simulink model "HDVPSG_DelayComp_NewRef_RealDrop_case1"  (R2019b)
settings: Solver=FixedStepDiscrete  StartTime=0.0  StopTime=28  FixedStep=UT.Ts_Veh  RelTol=1e-3
PostLoadFcn:
  | if any(exist('dsrtsu_mdlpostloadfcn', 'file') ~= 0), dsrtsu_mdlpostloadfcn('Execute', bdroot); end
InitFcn:
  | , if any(exist('dsmpb_private', 'file') ~= 0), dsmpb_private('dsmpb_mdlclblib', 'Init', bdroot); end,
values from neighbouring files (symbols this model uses):
  BETA_HDV_Leader = 50    [HDVPSG_DelayComp_NewRef_RealDrop_script_case1.m]
  BETA_PSG_Follower = 150    [HDVPSG_DelayComp_NewRef_RealDrop_script_case1.m]
  CtrlZone_Length = 250    [HDVPSG_DelayComp_NewRef_RealDrop_script_case1.m]
  DELTA_D_MIN = 5    [HDVPSG_DelayComp_NewRef_RealDrop_script_case1.m]
  DELTA_DR_MG_TCC = 15    [HDVPSG_DelayComp_NewRef_RealDrop_script_case1.m]
  HDV_AMAX = 1.3    [HDVPSG_DelayComp_NewRef_RealDrop_script_case1.m]
  HDV_AMIN = -2.5    [HDVPSG_DelayComp_NewRef_RealDrop_script_case1.m]
  HDV_first_v0 = 13    [HDVPSG_DelayComp_NewRef_RealDrop_script_case1.m]
  HDV_HighMu_D = 9    [HDVPSG_DelayComp_NewRef_RealDrop_script_case1.m]
  HDV_HighMu_I = 27    [HDVPSG_DelayComp_NewRef_RealDrop_script_case1.m]
  HDV_HighMu_P = 27    [HDVPSG_DelayComp_NewRef_RealDrop_script_case1.m]
  HDV_HighMu_TRFC = 0.7    [HDVPSG_DelayComp_NewRef_RealDrop_script_case1.m]
  HDV_last_v0 = 13    [HDVPSG_DelayComp_NewRef_RealDrop_script_case1.m]
  HDV_LowMu_D = 6    [HDVPSG_DelayComp_NewRef_RealDrop_script_case1.m]
  HDV_LowMu_I = 8    [HDVPSG_DelayComp_NewRef_RealDrop_script_case1.m]
  HDV_LowMu_P = 12    [HDVPSG_DelayComp_NewRef_RealDrop_script_case1.m]
  HDV_LowMu_TRFC = 0.6    [HDVPSG_DelayComp_NewRef_RealDrop_script_case1.m]
  Np_MPC = 20    [HDVPSG_DelayComp_NewRef_RealDrop_script_case1.m]
  PSG_AMAX = 3.2    [HDVPSG_DelayComp_NewRef_RealDrop_script_case1.m]
  PSG_AMIN = -6    [HDVPSG_DelayComp_NewRef_RealDrop_script_case1.m]
  PSG_end_v0 = 13    [HDVPSG_DelayComp_NewRef_RealDrop_script_case1.m]
  PSG_first_v0 = 13    [HDVPSG_DelayComp_NewRef_RealDrop_script_case1.m]
  PSG_HighMu_D = 15    [HDVPSG_DelayComp_NewRef_RealDrop_script_case1.m]
  PSG_HighMu_I = 125    [HDVPSG_DelayComp_NewRef_RealDrop_script_case1.m]
  PSG_HighMu_P = 75    [HDVPSG_DelayComp_NewRef_RealDrop_script_case1.m]
  PSG_HighMu_TRFC = 0.8    [HDVPSG_DelayComp_NewRef_RealDrop_script_case1.m]
  PSG_LowMu_D = 12    [HDVPSG_DelayComp_NewRef_RealDrop_script_case1.m]
  PSG_LowMu_I = 64    [HDVPSG_DelayComp_NewRef_RealDrop_script_case1.m]
  PSG_LowMu_P = 48    [HDVPSG_DelayComp_NewRef_RealDrop_script_case1.m]
  PSG_LowMu_TRFC = 0.7    [HDVPSG_DelayComp_NewRef_RealDrop_script_case1.m]
  PSG_middle_v0 = 13    [HDVPSG_DelayComp_NewRef_RealDrop_script_case1.m]
  Q_Leader = 1    [HDVPSG_DelayComp_NewRef_RealDrop_script_case1.m]
  Qd_dot_PSG_Follower = 2    [HDVPSG_DelayComp_NewRef_RealDrop_script_case1.m]
  Qd_PSG_Follower = 10    [HDVPSG_DelayComp_NewRef_RealDrop_script_case1.m]
  R_Leader = 20    [HDVPSG_DelayComp_NewRef_RealDrop_script_case1.m]
  R_PSG_Follower = 1    [HDVPSG_DelayComp_NewRef_RealDrop_script_case1.m]
  Recved_40_1 = Recved_Flag_Combined(47740,:)    [HDVPSG_DelayComp_NewRef_RealDrop_script_case1.m]
  Recved_40_2 = Recved_Flag_Combined(47780,:)    [HDVPSG_DelayComp_NewRef_RealDrop_script_case1.m]
  Recved_40_3 = Recved_Flag_Combined(49536,:)    [HDVPSG_DelayComp_NewRef_RealDrop_script_case1.m]
  Recved_40_4 = Recved_Flag_Combined(118106,:)    [HDVPSG_DelayComp_NewRef_RealDrop_script_case1.m]
  Rho_deltad_PSG_Follower = 1e3    (= 1000)    [HDVPSG_DelayComp_NewRef_RealDrop_script_case1.m]
  Rho_v_PSG_Follower = 1e3    (= 1000)    [HDVPSG_DelayComp_NewRef_RealDrop_script_case1.m]
  T_ADE = 0.01    [HDVPSG_DelayComp_NewRef_RealDrop_script_case1.m]
  V_MAX = 40    [HDVPSG_DelayComp_NewRef_RealDrop_script_case1.m]
  V_MIN = 0    [HDVPSG_DelayComp_NewRef_RealDrop_script_case1.m]
  VR_MG_TCC = 15    [HDVPSG_DelayComp_NewRef_RealDrop_script_case1.m]
undefined symbols (not defined in the file or in its folder): DiscIntNeverNeededParam, UT
libraries: simulink x46
(part 14 of 16)

== system HDVPSG_DelayComp_NewRef_RealDrop_case1/Subsystem6/HDV_first/Body Fixed Vehicle Dynamics/8dof_vehicle/longitudinal ==
  In1 : Inport
  In2 : Inport  Port=2
  In5 : Inport  Port=3
  In6 : Inport  Port=4
  In3 : Inport  Port=5
  In4 : Inport  Port=6
  Fax : Inport  Port=7
  Fr : Inport  Port=8
  slope : Inport  Port=9
  Vy : Inport  Port=10
  deltaFL : Inport  Port=11
  deltaFR : Inport  Port=12
  pitch : Inport  Port=13
  pitch_rate : Inport  Port=14
  pitch_accel : Inport  Port=15
  roll : Inport  Port=16
  roll_rate : Inport  Port=17
  roll_accel : Inport  Port=18
  yaw_rate : Inport  Port=19
  yaw_accel : Inport  Port=20
  V_ini : Inport  Port=21
  Add : Sum  Inputs=+-++---
  Add1 : Sum  Inputs=+++
  Add2 : Sum
  Add3 : Sum  Inputs=+++
  Add4 : Sum
  Add5 : Sum  Inputs=+---++
  Constant : Constant  Value=UT.Mv
  Constant1 : Constant  Value=UT.g
  Discrete-Time Integrator : DiscreteIntegrator  InitialConditionSource=external  InitialCondition=UT.Veh_PSG_o(1)  SampleTime=UT.Ts_Veh  ICPrevOutput=DiscIntNeverNeededParam  ICPrevScaledInput=DiscIntNeverNeededParam
  Gain : Gain  Gain=1/UT.Mv
  Gain1 : Gain  Gain=UT.h
  Gain2 : Gain
  Gain3 : Gain  Gain=2
  Gain4 : Gain  Gain=2
  Math Function : Math  Operator=square  SaturateOnIntegerOverflow=on
  Math Function1 : Math  Operator=square  SaturateOnIntegerOverflow=on
  Math Function2 : Math  Operator=square  SaturateOnIntegerOverflow=on
  Product{,1..2,4..5,7} (6 alike) : Product
  Product10 : Product  Inputs=4
  Product{3,6,8..9,11} (5 alike) : Product  Inputs=3
  Saturation : Saturate  UpperLimit=50  LowerLimit=0
  Trigonometric {,3,6..7} (4 alike) : Trigonometry  Operator=cos
  Trigonometric {1..2,4..5,8} (5 alike) : Trigonometry
  yaw_rate1 : InportShadow  Port=19
  ax : Outport  VectorParamsAs1DForOutWhenUnconnected=off
  Vx : Outport  Port=2  VectorParamsAs1DForOutWhenUnconnected=off
  Fx : Outport  Port=3  VectorParamsAs1DForOutWhenUnconnected=off
  wires:
  Add5/1 -> Gain1/1
  roll_accel/1 -> Product11/3
  Product11/1 -> Add5/6
  Trigonometric 8/1 -> Product10/2, Product11/1
  Product10/1 -> Gain4/1
  Gain4/1 -> Add5/5
  Product9/1 -> Add5/4
  pitch_accel/1 -> Product9/3
  Trigonometric 7/1 -> Product9/2, Product10/1
  Gain3/1 -> Add5/3
  Product8/1 -> Gain3/1
  Product7/1 -> Add5/2
  yaw_accel/1 -> Product7/2
  Product6/1 -> Add5/1
  Trigonometric 5/1 -> Product6/1, Product11/2, Product7/1
  Trigonometric 6/1 -> Product6/2, Product8/1, Product9/1
  roll/1 -> Trigonometric 6/1, Trigonometric 8/1
  pitch/1 -> Trigonometric 5/1, Trigonometric 7/1
  Add3/1 -> Product6/3
  Math Function2/1 -> Add3/3
  Math Function1/1 -> Add3/2
  Math Function/1 -> Add3/1
  yaw_rate/1 -> Math Function2/1, Product8/3
  roll_rate/1 -> Math Function1/1, Product8/2, Product10/3
  pitch_rate/1 -> Math Function/1, Product10/4
  Gain1/1 -> Add1/3
  Saturation/1 -> Vx/1
  Product5/1 -> Add2/2
  Product2/1 -> Add2/1
  Trigonometric 4/1 -> Product5/2
  Trigonometric 1/1 -> Product2/2
  Trigonometric 3/1 -> Product1/2
  deltaFR/1 -> Trigonometric 3/1, Trigonometric 4/1
  "Trigonometric "/1 -> Product4/2
  deltaFL/1 -> "Trigonometric "/1, Trigonometric 1/1
  In2/1 -> Product1/1
  Product1/1 -> Add4/2
  Gain2/1 -> Add/6
  Constant/1 -> Product3/2
  Constant1/1 -> Product3/1
  Trigonometric 2/1 -> Product3/3
  Add1/1 -> ax/1, Discrete-Time Integrator/1
  In6/1 -> Add/4
  In5/1 -> Add/3
  Add2/1 -> Add/2
  In4/1 -> Product5/1
  In3/1 -> Product2/1
  Add4/1 -> Add/1
  Product4/1 -> Add4/1
  In1/1 -> Product4/1
  Gain/1 -> Add1/1
  Product/1 -> Add1/2
  Add/1 -> Gain/1, Fx/1
  Vy/1 -> Product/2
  yaw_rate1/1 -> Product/1
  Product3/1 -> Add/7
  slope/1 -> Trigonometric 2/1
  Fr/1 -> Gain2/1
  Fax/1 -> Add/5
  Discrete-Time Integrator/1 -> Saturation/1
  V_ini/1 -> Discrete-Time Integrator/2

== system HDVPSG_DelayComp_NewRef_RealDrop_case1/Subsystem6/HDV_first/Body Fixed Vehicle Dynamics/Driving Resistance Subsystem/Aerodynamic Resistance ==
  note: increaesd to 0.75*...
  note: Vx=m/s
  note: Fa=0.5*p*Cd*A(Vx+Vw)^2
  Vx : Inport
  X Aerodynamic Fcn : Fcn  Expr=0.75*UT.rho*UT.Cd*UT.Awind*(u(1)+UT.Vw)^2  SampleTime=UT.Ts_Veh
  Fa : Outport  VectorParamsAs1DForOutWhenUnconnected=off
  wires:
  Vx/1 -> X Aerodynamic Fcn/1
  X Aerodynamic Fcn/1 -> Fa/1

== system HDVPSG_DelayComp_NewRef_RealDrop_case1/Subsystem6/HDV_first/Body Fixed Vehicle Dynamics/Driving Resistance Subsystem/Rolling resistance ==
  note: added *2
  Vx : Inport
  Rolling resistance Fcn1 : Fcn  Expr=(0.005+(1/2.013)*(0.01+0.0095*((3.6*u(1))/100)^2))*UT.Mv*UT.g*2  SampleTime=UT.Ts_Veh
  Fr : Outport  VectorParamsAs1DForOutWhenUnconnected=off
  wires:
  Rolling resistance Fcn1/1 -> Fr/1
  Vx/1 -> Rolling resistance Fcn1/1

== system HDVPSG_DelayComp_NewRef_RealDrop_case1/Subsystem6/HDV_first/Body Fixed Vehicle Dynamics/Fz/FZ FL ==
  note: 0.5
  ax : Inport
  slope : Inport  Port=2
  ay : Inport  Port=3
  bank : Inport  Port=4
  Fa : Inport  Port=5
  Add1 : Sum  Inputs=--+-+-+
  Constant : Constant  Value=UT.ha
  Constant1 : Constant  Value=UT.Ms
  Constant{3,10,17,23} (4 alike) : Constant  Value=UT.g
  Constant11 : Constant  Value=UT.lf+UT.lr
  Constant{8,12,15,20} (4 alike) : Constant  Value=UT.Mv
  Constant{2,6,9,13} (4 alike) : Constant  Value=UT.h
  Constant14 : Constant  Value=2*UT.Ls
  Constant16 : Constant  Value=UT.lr
  Constant18 : Constant  Value=UT.lf +UT.lr
  Constant19 : Constant  Value=UT.lf+UT.lr
  Constant21 : Constant  Value=UT.Ls
  Constant22 : Constant  Value=2*UT.Ls
  Constant4 : Constant  Value=UT.lf+UT.lr
  Constant5 : Constant  Value=UT.Ms
  Constant7 : Constant  Value=2*UT.Ls
  Divide{,1..6} (7 alike) : Product  Inputs=*/
  Gain{,1..6} (7 alike) : Gain  Gain=0.25
  Product : Product
  Product1 : Product  Inputs=3
  Product{2,4..6} (4 alike) : Product  Inputs=4
  Product3 : Product  Inputs=3
  Trigonometric Function : Trigonometry
  Trigonometric Function1 : Trigonometry
  Trigonometric Function2 : Trigonometry  Operator=cos
  Trigonometric Function3 : Trigonometry  Operator=cos
  bank1 : InportShadow  Port=4
  slope1 : InportShadow  Port=2
  Out1 : Outport  VectorParamsAs1DForOutWhenUnconnected=off
  wires:
  Gain6/1 -> Add1/7
  Divide6/1 -> Gain6/1
  Constant22/1 -> Divide6/2
  Product6/1 -> Divide6/1
  Trigonometric Function3/1 -> Product6/4
  bank1/1 -> Trigonometric Function3/1
  Constant23/1 -> Product6/3
  Constant21/1 -> Product6/2
  Constant20/1 -> Product6/1
  Gain2/1 -> Add1/6
  Gain4/1 -> Add1/3
  Gain3/1 -> Add1/5
  Gain1/1 -> Add1/4
  Gain/1 -> Add1/2
  Gain5/1 -> Add1/1
  Divide5/1 -> Gain5/1
  Constant19/1 -> Divide5/2
  Product/1 -> Divide5/1
  Constant/1 -> Product/2
  Fa/1 -> Product/1
  Product1/1 -> Divide/1
  Add1/1 -> Out1/1
  Divide4/1 -> Gain3/1
  Product5/1 -> Divide4/1
  Constant18/1 -> Divide4/2
  slope1/1 -> Trigonometric Function2/1
  Trigonometric Function2/1 -> Product5/4
  Constant17/1 -> Product5/3
  Constant16/1 -> Product5/2
  Constant15/1 -> Product5/1
  Divide3/1 -> Gain2/1
  Constant14/1 -> Divide3/2
  Product2/1 -> Divide3/1
  Trigonometric Function1/1 -> Product2/4
  bank/1 -> Trigonometric Function1/1
  Constant3/1 -> Product2/3
  Constant13/1 -> Product2/2
  Constant12/1 -> Product2/1
  Product4/1 -> Divide2/1
  Divide2/1 -> Gain1/1
  Constant11/1 -> Divide2/2
  Trigonometric Function/1 -> Product4/4
  slope/1 -> Trigonometric Function/1
  Constant10/1 -> Product4/3
  Constant9/1 -> Product4/2
  Constant8/1 -> Product4/1
  Divide1/1 -> Gain4/1
  Divide/1 -> Gain/1
  Constant7/1 -> Divide1/2
  Product3/1 -> Divide1/1
  Constant6/1 -> Product3/3
  Constant5/1 -> Product3/2
  ay/1 -> Product3/1
  Constant4/1 -> Divide/2
  ax/1 -> Product1/3
  Constant2/1 -> Product1/2
  Constant1/1 -> Product1/1

== system HDVPSG_DelayComp_NewRef_RealDrop_case1/Subsystem6/HDV_first/Body Fixed Vehicle Dynamics/Fz/FZ FR ==
  note: 0.5
  ax : Inport
  slope : Inport  Port=2
  ay : Inport  Port=3
  bank : Inport  Port=4
  Fa : Inport  Port=5
  Add1 : Sum  Inputs=----+++
  Constant : Constant  Value=UT.ha
  Constant1 : Constant  Value=UT.Ms
  Constant{3,10,17,23} (4 alike) : Constant  Value=UT.g
  Constant{4,11,18..19} (4 alike) : Constant  Value=UT.lf+UT.lr
  Constant{8,12,15,20} (4 alike) : Constant  Value=UT.Mv
  Constant{2,6,9,13} (4 alike) : Constant  Value=UT.h
  Constant14 : Constant  Value=2*UT.Ls
  Constant16 : Constant  Value=UT.lr
  Constant21 : Constant  Value=UT.Ls
  Constant22 : Constant  Value=2*UT.Ls
  Constant5 : Constant  Value=UT.Ms
  Constant7 : Constant  Value=2*UT.Ls
  Divide{,1..6} (7 alike) : Product  Inputs=*/
  Gain{,1..6} (7 alike) : Gain  Gain=0.25
  Product : Product
  Product1 : Product  Inputs=3
  Product{2,4..6} (4 alike) : Product  Inputs=4
  Product3 : Product  Inputs=3
  Trigonometric Function : Trigonometry
  Trigonometric Function1 : Trigonometry
  Trigonometric Function2 : Trigonometry  Operator=cos
  Trigonometric Function3 : Trigonometry  Operator=cos
  bank1 : InportShadow  Port=4
  slope1 : InportShadow  Port=2
  Out1 : Outport  VectorParamsAs1DForOutWhenUnconnected=off
  wires:
  Constant1/1 -> Product1/1
  Constant2/1 -> Product1/2
  ax/1 -> Product1/3
  Constant4/1 -> Divide/2
  ay/1 -> Product3/1
  Constant5/1 -> Product3/2
  Constant6/1 -> Product3/3
  Product3/1 -> Divide1/1
  Constant7/1 -> Divide1/2
  Divide/1 -> Gain/1
  Divide1/1 -> Gain4/1
  Constant8/1 -> Product4/1
  Constant9/1 -> Product4/2
  Constant10/1 -> Product4/3
  slope/1 -> Trigonometric Function/1
  Trigonometric Function/1 -> Product4/4
  Constant11/1 -> Divide2/2
  Divide2/1 -> Gain1/1
  Product4/1 -> Divide2/1
  Constant12/1 -> Product2/1
  Constant13/1 -> Product2/2
  Constant3/1 -> Product2/3
  bank/1 -> Trigonometric Function1/1
  Trigonometric Function1/1 -> Product2/4
  Product2/1 -> Divide3/1
  Constant14/1 -> Divide3/2
  Divide3/1 -> Gain2/1
  Constant15/1 -> Product5/1
  Constant16/1 -> Product5/2
  Constant17/1 -> Product5/3
  Trigonometric Function2/1 -> Product5/4
  slope1/1 -> Trigonometric Function2/1
  Constant18/1 -> Divide4/2
  Product5/1 -> Divide4/1
  Divide4/1 -> Gain3/1
  Add1/1 -> Out1/1
  Product1/1 -> Divide/1
  Fa/1 -> Product/1
  Constant/1 -> Product/2
  Product/1 -> Divide5/1
  Constant19/1 -> Divide5/2
  Divide5/1 -> Gain5/1
  Gain5/1 -> Add1/1
  Gain/1 -> Add1/2
  Gain1/1 -> Add1/4
  Gain3/1 -> Add1/5
  Gain4/1 -> Add1/3
  Gain2/1 -> Add1/6
  Constant20/1 -> Product6/1
  Constant21/1 -> Product6/2
  Constant23/1 -> Product6/3
  bank1/1 -> Trigonometric Function3/1
  Trigonometric Function3/1 -> Product6/4
  Product6/1 -> Divide6/1
  Constant22/1 -> Divide6/2
  Divide6/1 -> Gain6/1
  Gain6/1 -> Add1/7

== system HDVPSG_DelayComp_NewRef_RealDrop_case1/Subsystem6/HDV_first/Body Fixed Vehicle Dynamics/Fz/FZ RL ==
  note: 0.5
  ax : Inport
  slope : Inport  Port=2
  ay : Inport  Port=3
  bank : Inport  Port=4
  Fa : Inport  Port=5
  Add1 : Sum  Inputs=+++++-+
  Constant : Constant  Value=UT.ha
  Constant1 : Constant  Value=UT.Ms
  Constant{3,10,17,23} (4 alike) : Constant  Value=UT.g
  Constant{4,11,18..19} (4 alike) : Constant  Value=UT.lf+UT.lr
  Constant{8,12,15,20} (4 alike) : Constant  Value=UT.Mv
  Constant{2,6,9,13} (4 alike) : Constant  Value=UT.h
  Constant14 : Constant  Value=2*UT.Ls
  Constant16 : Constant  Value=UT.lf
  Constant21 : Constant  Value=UT.Ls
  Constant22 : Constant  Value=2*UT.Ls
  Constant5 : Constant  Value=UT.Ms
  Constant7 : Constant  Value=2*UT.Ls
  Divide{,1..6} (7 alike) : Product  Inputs=*/
  Gain{,1..6} (7 alike) : Gain  Gain=0.25
  Product : Product
  Product1 : Product  Inputs=3
  Product{2,4..6} (4 alike) : Product  Inputs=4
  Product3 : Product  Inputs=3
  Trigonometric Function : Trigonometry
  Trigonometric Function1 : Trigonometry
  Trigonometric Function2 : Trigonometry  Operator=cos
  Trigonometric Function3 : Trigonometry  Operator=cos
  bank1 : InportShadow  Port=4
  slope1 : InportShadow  Port=2
  Out1 : Outport  VectorParamsAs1DForOutWhenUnconnected=off
  wires:
  Constant1/1 -> Product1/1
  Constant2/1 -> Product1/2
  ax/1 -> Product1/3
  Constant4/1 -> Divide/2
  ay/1 -> Product3/1
  Constant5/1 -> Product3/2
  Constant6/1 -> Product3/3
  Product3/1 -> Divide1/1
  Constant7/1 -> Divide1/2
  Divide/1 -> Gain/1
  Divide1/1 -> Gain4/1
  Constant8/1 -> Product4/1
  Constant9/1 -> Product4/2
  Constant10/1 -> Product4/3
  slope/1 -> Trigonometric Function/1
  Trigonometric Function/1 -> Product4/4
  Constant11/1 -> Divide2/2
  Divide2/1 -> Gain1/1
  Product4/1 -> Divide2/1
  Constant12/1 -> Product2/1
  Constant13/1 -> Product2/2
  Constant3/1 -> Product2/3
  bank/1 -> Trigonometric Function1/1
  Trigonometric Function1/1 -> Product2/4
  Product2/1 -> Divide3/1
  Constant14/1 -> Divide3/2
  Divide3/1 -> Gain2/1
  Constant15/1 -> Product5/1
  Constant16/1 -> Product5/2
  Constant17/1 -> Product5/3
  Trigonometric Function2/1 -> Product5/4
  slope1/1 -> Trigonometric Function2/1
  Constant18/1 -> Divide4/2
  Product5/1 -> Divide4/1
  Divide4/1 -> Gain3/1
  Add1/1 -> Out1/1
  Product1/1 -> Divide/1
  Fa/1 -> Product/1
  Constant/1 -> Product/2
  Product/1 -> Divide5/1
  Constant19/1 -> Divide5/2
  Divide5/1 -> Gain5/1
  Gain5/1 -> Add1/1
  Gain/1 -> Add1/2
  Gain1/1 -> Add1/4
  Gain3/1 -> Add1/5
  Gain4/1 -> Add1/3
  Gain2/1 -> Add1/6
  Constant20/1 -> Product6/1
  Constant21/1 -> Product6/2
  Constant23/1 -> Product6/3
  bank1/1 -> Trigonometric Function3/1
  Trigonometric Function3/1 -> Product6/4
  Product6/1 -> Divide6/1
  Constant22/1 -> Divide6/2
  Divide6/1 -> Gain6/1
  Gain6/1 -> Add1/7

== system HDVPSG_DelayComp_NewRef_RealDrop_case1/Subsystem6/HDV_first/Body Fixed Vehicle Dynamics/Fz/FZ RR ==
  note: 0.5
  ax : Inport
  slope : Inport  Port=2
  ay : Inport  Port=3
  bank : Inport  Port=4
  Fa : Inport  Port=5
  Add1 : Sum  Inputs=++-++++
  Constant : Constant  Value=UT.ha
  Constant1 : Constant  Value=UT.Ms
  Constant{3,10,17,23} (4 alike) : Constant  Value=UT.g
  Constant{4,11,18..19} (4 alike) : Constant  Value=UT.lf+UT.lr
  Constant{8,12,15,20} (4 alike) : Constant  Value=UT.Mv
  Constant{2,6,9,13} (4 alike) : Constant  Value=UT.h
  Constant14 : Constant  Value=2*UT.Ls
  Constant16 : Constant  Value=UT.lf
  Constant21 : Constant  Value=UT.Ls
  Constant22 : Constant  Value=2*UT.Ls
  Constant5 : Constant  Value=UT.Ms
  Constant7 : Constant  Value=2*UT.Ls
  Divide{,1..6} (7 alike) : Product  Inputs=*/
  Gain{,1..6} (7 alike) : Gain  Gain=0.25
  Product : Product
  Product1 : Product  Inputs=3
  Product{2,4..6} (4 alike) : Product  Inputs=4
  Product3 : Product  Inputs=3
  Trigonometric Function : Trigonometry
  Trigonometric Function1 : Trigonometry
  Trigonometric Function2 : Trigonometry  Operator=cos
  Trigonometric Function3 : Trigonometry  Operator=cos
  bank1 : InportShadow  Port=4
  slope1 : InportShadow  Port=2
  Out1 : Outport  VectorParamsAs1DForOutWhenUnconnected=off
  wires:
  Gain6/1 -> Add1/7
  Divide6/1 -> Gain6/1
  Constant22/1 -> Divide6/2
  Product6/1 -> Divide6/1
  Trigonometric Function3/1 -> Product6/4
  bank1/1 -> Trigonometric Function3/1
  Constant23/1 -> Product6/3
  Constant21/1 -> Product6/2
  Constant20/1 -> Product6/1
  Gain2/1 -> Add1/6
  Gain4/1 -> Add1/3
  Gain3/1 -> Add1/5
  Gain1/1 -> Add1/4
  Gain/1 -> Add1/2
  Gain5/1 -> Add1/1
  Divide5/1 -> Gain5/1
  Constant19/1 -> Divide5/2
  Product/1 -> Divide5/1
  Constant/1 -> Product/2
  Fa/1 -> Product/1
  Product1/1 -> Divide/1
  Add1/1 -> Out1/1
  Divide4/1 -> Gain3/1
  Product5/1 -> Divide4/1
  Constant18/1 -> Divide4/2
  slope1/1 -> Trigonometric Function2/1
  Trigonometric Function2/1 -> Product5/4
  Constant17/1 -> Product5/3
  Constant16/1 -> Product5/2
  Constant15/1 -> Product5/1
  Divide3/1 -> Gain2/1
  Constant14/1 -> Divide3/2
  Product2/1 -> Divide3/1
  Trigonometric Function1/1 -> Product2/4
  bank/1 -> Trigonometric Function1/1
  Constant3/1 -> Product2/3
  Constant13/1 -> Product2/2
  Constant12/1 -> Product2/1
  Product4/1 -> Divide2/1
  Divide2/1 -> Gain1/1
  Constant11/1 -> Divide2/2
  Trigonometric Function/1 -> Product4/4
  slope/1 -> Trigonometric Function/1
  Constant10/1 -> Product4/3
  Constant9/1 -> Product4/2
  Constant8/1 -> Product4/1
  Divide1/1 -> Gain4/1
  Divide/1 -> Gain/1
  Constant7/1 -> Divide1/2
  Product3/1 -> Divide1/1
  Constant6/1 -> Product3/3
  Constant5/1 -> Product3/2
  ay/1 -> Product3/1
  Constant4/1 -> Divide/2
  ax/1 -> Product1/3
  Constant2/1 -> Product1/2
  Constant1/1 -> Product1/1

== matlab function HDVPSG_DelayComp_NewRef_RealDrop_case1/ARE_First_Order_Derivative_[1,0,0]1/MATLAB Function ==
  data: U input; Dot_U output; Ts input; u_init input
function Dot_U = buffer(U, Ts, u_init)
    N = 12;
    %Ts = 0.01;
    persistent y;
    if isempty(y)
        y=u_init*ones(N+1,1);%m/s
    end

    y = [U;y(1:end-1)];
    T = Ts*N;
    P = zeros(1,N+1);
    P_alpha = P;
    for k = 1:N+1
        tao_k = (k-1)*Ts;
        P(k) = T-2*tao_k;
        if((k==1)||(k==N+1))
            P_alpha(k) = P(k)*Ts/2;
        else
            P_alpha(k) = P(k)*Ts;
        end
    end
    
    Dot_U = P_alpha*y*6/(T^3);

end

== matlab function HDVPSG_DelayComp_NewRef_RealDrop_case1/ARE_First_Order_Derivative_[1,0,0]2/MATLAB Function ==
  data: U input; Dot_U output; Ts input; u_init input
function Dot_U = buffer(U, Ts, u_init)
    N = 12;
    %Ts = 0.01;
    persistent y;
    if isempty(y)
        y=u_init*ones(N+1,1);%m/s
    end

    y = [U;y(1:end-1)];
    T = Ts*N;
    P = zeros(1,N+1);
    P_alpha = P;
    for k = 1:N+1
        tao_k = (k-1)*Ts;
        P(k) = T-2*tao_k;
        if((k==1)||(k==N+1))
            P_alpha(k) = P(k)*Ts/2;
        else
            P_alpha(k) = P(k)*Ts;
        end
    end
    
    Dot_U = P_alpha*y*6/(T^3);

end

== matlab function HDVPSG_DelayComp_NewRef_RealDrop_case1/ARE_First_Order_Derivative_[1,0,0]4/MATLAB Function ==
  data: U input; Dot_U output; Ts input; u_init input
function Dot_U = buffer(U, Ts, u_init)
    N = 12;
    %Ts = 0.01;
    persistent y;
    if isempty(y)
        y=u_init*ones(N+1,1);%m/s
    end

    y = [U;y(1:end-1)];
    T = Ts*N;
    P = zeros(1,N+1);
    P_alpha = P;
    for k = 1:N+1
        tao_k = (k-1)*Ts;
        P(k) = T-2*tao_k;
        if((k==1)||(k==N+1))
            P_alpha(k) = P(k)*Ts/2;
        else
            P_alpha(k) = P(k)*Ts;
        end
    end
    
    Dot_U = P_alpha*y*6/(T^3);

end

== matlab function HDVPSG_DelayComp_NewRef_RealDrop_case1/ARE_First_Order_Derivative_[1,0,0]5/MATLAB Function ==
  data: U input; Dot_U output; Ts input; u_init input
function Dot_U = buffer(U, Ts, u_init)
    N = 12;
    %Ts = 0.01;
    persistent y;
    if isempty(y)
        y=u_init*ones(N+1,1);%m/s
    end

    y = [U;y(1:end-1)];
    T = Ts*N;
    P = zeros(1,N+1);
    P_alpha = P;
    for k = 1:N+1
        tao_k = (k-1)*Ts;
        P(k) = T-2*tao_k;
        if((k==1)||(k==N+1))
            P_alpha(k) = P(k)*Ts/2;
        else
            P_alpha(k) = P(k)*Ts;
        end
    end
    
    Dot_U = P_alpha*y*6/(T^3);

end

== matlab function HDVPSG_DelayComp_NewRef_RealDrop_case1/PSG2_control_withPDR_compen/MATLAB Function ==
  data: REALWORLD_DIST output; X_Ego input; Rho_delta_d_adpt output; Y_Ego input; X_Front input; Y_Front input; DELTA_D_MIN input; Rho_delta_dMAX input
function [REALWORLD_DIST, Rho_delta_d_adpt] = Adaptive_Rho_delta_d(X_Ego, Y_Ego, X_Front, Y_Front, DELTA_D_MIN, Rho_delta_dMAX)
    REALWORLD_DIST = sqrt((X_Ego - X_Front)^2 + (Y_Ego - Y_Front)^2); % The virtual leading car may be in another lane: So far away from the ego_car

    if REALWORLD_DIST>2*DELTA_D_MIN  %  This is determined by the road geometry
        Rho_delta_d_adpt = 0; % Disable 
    elseif REALWORLD_DIST>DELTA_D_MIN
        Rho_delta_d_adpt = -Rho_delta_dMAX/DELTA_D_MIN*REALWORLD_DIST + 2*Rho_delta_dMAX;   % linear adaptive gain
    else
        Rho_delta_d_adpt = Rho_delta_dMAX;
    end
    
end

== matlab function HDVPSG_DelayComp_NewRef_RealDrop_case1/leader_ulmpc_spd_ctrl/Optimal_Control_Reference ==
  data: L_ctz input; opt_pos output; v_ini input; a_ini input; v_mp input; T_rest_to_MP input; t_aft_trigger input; opt_spd output; opt_acc output; opt_pos_vec output; opt_spd_vec output; alpha output; beta output; c_1 output; c_2 output; c_3 output; c_4 output
function [opt_pos, opt_spd, opt_acc, opt_pos_vec, opt_spd_vec, alpha, beta, c_1, c_2, c_3, c_4] = Opt_Ref(L_ctz, v_ini, a_ini, v_mp, T_rest_to_MP, t_aft_trigger)
Np          = 20;
opt_pos_vec = zeros(1, Np+1);
opt_spd_vec = zeros(1, Np+1);
%opt_acc_vec = zeros(1, Np+1);

Ts    = 0.01;
L_ctz = -L_ctz;

alpha = -(12*v_mp - 12*v_ini - 12*L_ctz - 6*T_rest_to_MP*a_ini - 12*T_rest_to_MP*v_mp + 6*T_rest_to_MP*L_ctz + 2*T_rest_to_MP^2*a_ini + 2*T_rest_to_MP^2*v_ini + 4*T_rest_to_MP^2*v_mp + 12*v_ini*exp(-T_rest_to_MP) - 12*v_mp*exp(-T_rest_to_MP) + 12*L_ctz*exp(-T_rest_to_MP) + 6*T_rest_to_MP*a_ini*exp(-T_rest_to_MP) + 12*T_rest_to_MP*v_ini*exp(-T_rest_to_MP) + 6*T_rest_to_MP*L_ctz*exp(-T_rest_to_MP) + 4*T_rest_to_MP^2*a_ini*exp(-T_rest_to_MP) + T_rest_to_MP^3*a_ini*exp(-T_rest_to_MP) + 4*T_rest_to_MP^2*v_ini*exp(-T_rest_to_MP) + 2*T_rest_to_MP^2*v_mp*exp(-T_rest_to_MP))/(24*exp(-T_rest_to_MP) + 24*exp(T_rest_to_MP) + 8*T_rest_to_MP^2*exp(-T_rest_to_MP) + T_rest_to_MP^3*exp(-T_rest_to_MP) - 24*T_rest_to_MP*exp(T_rest_to_MP) + 8*T_rest_to_MP^2 + 24*T_rest_to_MP*exp(-T_rest_to_MP) + 8*T_rest_to_MP^2*exp(T_rest_to_MP) - T_rest_to_MP^3*exp(T_rest_to_MP) - 48);

beta  = -(12*v_mp - 12*v_ini + 12*L_ctz - 6*T_rest_to_MP*a_ini + 12*T_rest_to_MP*v_mp + 6*T_rest_to_MP*L_ctz - 2*T_rest_to_MP^2*a_ini + 2*T_rest_to_MP^2*v_ini + 4*T_rest_to_MP^2*v_mp + 12*v_ini*exp(T_rest_to_MP) - 12*v_mp*exp(T_rest_to_MP) - 12*L_ctz*exp(T_rest_to_MP) - 4*T_rest_to_MP^2*a_ini*exp(T_rest_to_MP) + T_rest_to_MP^3*a_ini*exp(T_rest_to_MP) + 4*T_rest_to_MP^2*v_ini*exp(T_rest_to_MP) + 2*T_rest_to_MP^2*v_mp*exp(T_rest_to_MP) + 6*T_rest_to_MP*a_ini*exp(T_rest_to_MP) - 12*T_rest_to_MP*v_ini*exp(T_rest_to_MP) + 6*T_rest_to_MP*L_ctz*exp(T_rest_to_MP))/(24*exp(-T_rest_to_MP) + 24*exp(T_rest_to_MP) + 8*T_rest_to_MP^2*exp(-T_rest_to_MP) + T_rest_to_MP^3*exp(-T_rest_to_MP) - 24*T_rest_to_MP*exp(T_rest_to_MP) + 8*T_rest_to_MP^2 + 24*T_rest_to_MP*exp(-T_rest_to_MP) + 8*T_rest_to_MP^2*exp(T_rest_to_MP) - T_rest_to_MP^3*exp(T_rest_to_MP) - 48);

  c_1 = -(6*(8*L_ctz - 8*a_ini + 4*T_rest_to_MP*v_ini + 4*T_rest_to_MP*v_mp + 2*T_rest_to_MP^2*a_ini + 4*a_ini*exp(T_rest_to_MP) - 4*L_ctz*exp(T_rest_to_MP) + 4*a_ini*exp(-T_rest_to_MP) - 4*L_ctz*exp(-T_rest_to_MP) + 4*T_rest_to_MP*a_ini*exp(-T_rest_to_MP) + T_rest_to_MP^2*a_ini*exp(T_rest_to_MP) - 2*T_rest_to_MP*v_ini*exp(-T_rest_to_MP) + T_rest_to_MP^2*v_ini*exp(T_rest_to_MP) - 2*T_rest_to_MP*v_mp*exp(-T_rest_to_MP) + T_rest_to_MP^2*v_mp*exp(T_rest_to_MP) - 2*T_rest_to_MP*L_ctz*exp(-T_rest_to_MP) + T_rest_to_MP^2*a_ini*exp(-T_rest_to_MP) - T_rest_to_MP^2*v_ini*exp(-T_rest_to_MP) - T_rest_to_MP^2*v_mp*exp(-T_rest_to_MP) - 4*T_rest_to_MP*a_ini*exp(T_rest_to_MP) - 2*T_rest_to_MP*v_ini*exp(T_rest_to_MP) - 2*T_rest_to_MP*v_mp*exp(T_rest_to_MP) + 2*T_rest_to_MP*L_ctz*exp(T_rest_to_MP)))/(T_rest_to_MP*(24*exp(-T_rest_to_MP) + 24*exp(T_rest_to_MP) + 8*T_rest_to_MP^2*exp(-T_rest_to_MP) + T_rest_to_MP^3*exp(-T_rest_to_MP) - 24*T_rest_to_MP*exp(T_rest_to_MP) + 8*T_rest_to_MP^2 + 24*T_rest_to_MP*exp(-T_rest_to_MP) + 8*T_rest_to_MP^2*exp(T_rest_to_MP) - T_rest_to_MP^3*exp(T_rest_to_MP) - 48)); 
  
  c_2 = (2*(12*L_ctz - 24*a_ini + 12*T_rest_to_MP*v_mp + 2*T_rest_to_MP^2*a_ini + 12*a_ini*exp(T_rest_to_MP) + 6*v_ini*exp(T_rest_to_MP) - 6*v_mp*exp(T_rest_to_MP) - 6*L_ctz*exp(T_rest_to_MP) + 12*a_ini*exp(-T_rest_to_MP) - 6*v_ini*exp(-T_rest_to_MP) + 6*v_mp*exp(-T_rest_to_MP) - 6*L_ctz*exp(-T_rest_to_MP) + 9*T_rest_to_MP*a_ini*exp(-T_rest_to_MP) + 2*T_rest_to_MP^2*a_ini*exp(T_rest_to_MP) - 6*T_rest_to_MP*v_ini*exp(-T_rest_to_MP) + 2*T_rest_to_MP^2*v_ini*exp(T_rest_to_MP) + T_rest_to_MP^2*v_mp*exp(T_rest_to_MP) - 3*T_rest_to_MP*L_ctz*exp(-T_rest_to_MP) + 2*T_rest_to_MP^2*a_ini*exp(-T_rest_to_MP) - 2*T_rest_to_MP^2*v_ini*exp(-T_rest_to_MP) - T_rest_to_MP^2*v_mp*exp(-T_rest_to_MP) - 9*T_rest_to_MP*a_ini*exp(T_rest_to_MP) - 6*T_rest_to_MP*v_ini*exp(T_rest_to_MP) + 3*T_rest_to_MP*L_ctz*exp(T_rest_to_MP)))/(24*exp(-T_rest_to_MP) + 24*exp(T_rest_to_MP) + 8*T_rest_to_MP^2*exp(-T_rest_to_MP) + T_rest_to_MP^3*exp(-T_rest_to_MP) - 24*T_rest_to_MP*exp(T_rest_to_MP) + 8*T_rest_to_MP^2 + 24*T_rest_to_MP*exp(-T_rest_to_MP) + 8*T_rest_to_MP^2*exp(T_rest_to_MP) - T_rest_to_MP^3*exp(T_rest_to_MP) - 48); 
  
  c_3 = -(24*v_ini + 24*v_mp - 12*T_rest_to_MP*a_ini + 12*T_rest_to_MP*L_ctz - 4*T_rest_to_MP^2*v_ini + 8*T_rest_to_MP^2*v_mp - 12*v_ini*exp(T_rest_to_MP) - 12*v_mp*exp(T_rest_to_MP) - 12*L_ctz*exp(T_rest_to_MP) - 12*v_ini*exp(-T_rest_to_MP) - 12*v_mp*exp(-T_rest_to_MP) + 12*L_ctz*exp(-T_rest_to_MP) + 6*T_rest_to_MP*a_ini*exp(-T_rest_to_MP) - 4*T_rest_to_MP^2*a_ini*exp(T_rest_to_MP) + T_rest_to_MP^3*a_ini*exp(T_rest_to_MP) - 12*T_rest_to_MP*v_ini*exp(-T_rest_to_MP) - 4*T_rest_to_MP^2*v_ini*exp(T_rest_to_MP) + T_rest_to_MP^3*v_ini*exp(T_rest_to_MP) + 2*T_rest_to_MP^2*v_mp*exp(T_rest_to_MP) + 6*T_rest_to_MP*L_ctz*exp(-T_rest_to_MP) + 4*T_rest_to_MP^2*a_ini*exp(-T_rest_to_MP) + T_rest_to_MP^3*a_ini*exp(-T_rest_to_MP) - 4*T_rest_to_MP^2*v_ini*exp(-T_rest_to_MP) - T_rest_to_MP^3*v_ini*exp(-T_rest_to_MP) + 2*T_rest_to_MP^2*v_mp*exp(-T_rest_to_MP) + 6*T_rest_to_MP*a_ini*exp(T_rest_to_MP) + 12*T_rest_to_MP*v_ini*exp(T_rest_to_MP) + 6*T_rest_to_MP*L_ctz*exp(T_rest_to_MP))/(24*exp(-T_rest_to_MP) + 24*exp(T_rest_to_MP) + 8*T_rest_to_MP^2*exp(-T_rest_to_MP) + T_rest_to_MP^3*exp(-T_rest_to_MP) - 24*T_rest_to_MP*exp(T_rest_to_MP) + 8*T_rest_to_MP^2 + 24*T_rest_to_MP*exp(-T_rest_to_MP) + 8*T_rest_to_MP^2*exp(T_rest_to_MP) - T_rest_to_MP^3*exp(T_rest_to_MP) - 48); 
  
  c_4 = -(24*L_ctz - 24*T_rest_to_MP*v_mp + 4*T_rest_to_MP^2*a_ini - 8*T_rest_to_MP^2*L_ctz - 12*v_ini*exp(T_rest_to_MP) + 12*v_mp*exp(T_rest_to_MP) - 12*L_ctz*exp(T_rest_to_MP) + 12*v_ini*exp(-T_rest_to_MP) - 12*v_mp*exp(-T_rest_to_MP) - 12*L_ctz*exp(-T_rest_to_MP) + 6*T_rest_to_MP*a_ini*exp(-T_rest_to_MP) + 4*T_rest_to_MP^2*a_ini*exp(T_rest_to_MP) - T_rest_to_MP^3*a_ini*exp(T_rest_to_MP) + 12*T_rest_to_MP*v_ini*exp(-T_rest_to_MP) - 4*T_rest_to_MP^2*v_ini*exp(T_rest_to_MP) - 2*T_rest_to_MP^2*v_mp*exp(T_rest_to_MP) - 18*T_rest_to_MP*L_ctz*exp(-T_rest_to_MP) - 8*T_rest_to_MP^2*L_ctz*exp(T_rest_to_MP) + T_rest_to_MP^3*L_ctz*exp(T_rest_to_MP) + 4*T_rest_to_MP^2*a_ini*exp(-T_rest_to_MP) + T_rest_to_MP^3*a_ini*exp(-T_rest_to_MP) + 4*T_rest_to_MP^2*v_ini*exp(-T_rest_to_MP) + 2*T_rest_to_MP^2*v_mp*exp(-T_rest_to_MP) - 8*T_rest_to_MP^2*L_ctz*exp(-T_rest_to_MP) - T_rest_to_MP^3*L_ctz*exp(-T_rest_to_MP) - 6*T_rest_to_MP*a_ini*exp(T_rest_to_MP) + 12*T_rest_to_MP*v_ini*exp(T_rest_to_MP) + 18*T_rest_to_MP*L_ctz*exp(T_rest_to_MP))/(24*exp(-T_rest_to_MP) + 24*exp(T_rest_to_MP) + 8*T_rest_to_MP^2*exp(-T_rest_to_MP) + T_rest_to_MP^3*exp(-T_rest_to_MP) - 24*T_rest_to_MP*exp(T_rest_to_MP) + 8*T_rest_to_MP^2 + 24*T_rest_to_MP*exp(-T_rest_to_MP) + 8*T_rest_to_MP^2*exp(T_rest_to_MP) - T_rest_to_MP^3*exp(T_rest_to_MP) - 48);
  
 % t = min(t, T_rest_to_MP);
  t_vec = t_aft_trigger + (1:(Np+1))*Ts;
 
 if t_aft_trigger <= T_rest_to_MP
     opt_pos = -alpha.*exp(t_aft_trigger) + beta.*exp(-t_aft_trigger) + 1/6.*c_1.*t_aft_trigger.^3 + c_2./2.*t_aft_trigger.^2 + c_3.*t_aft_trigger + c_4;
     opt_spd = -alpha.*exp(t_aft_trigger) - beta.*exp(-t_aft_trigger) + 1/2.*c_1.*t_aft_trigger.^2 + c_2.*t_aft_trigger + c_3;
     opt_acc = -alpha.*exp(t_aft_trigger) + beta.*exp(-t_aft_trigger) + c_1.*t_aft_trigger + c_2;
 else
     opt_pos = v_mp*(t_aft_trigger-T_rest_to_MP);
     opt_spd = v_mp;
     opt_acc = 0;
 end
 
for i = 1:Np+1
    if t_vec(i)<=T_rest_to_MP
        opt_pos_vec(i) = -alpha.*exp(t_vec(i)) + beta.*exp(-t_vec(i)) + 1/6.*c_1.*t_vec(i).^3 + c_2./2.*t_vec(i).^2 + c_3.*t_vec(i) + c_4;
        opt_spd_vec(i) = -alpha.*exp(t_vec(i)) - beta.*exp(-t_vec(i)) + 1/2.*c_1.*t_vec(i).^2 + c_2.*t_vec(i)       + c_3;
      %  opt_acc_vec(i) = -alpha.*exp(t_vec(i)) + beta.*exp(-t_vec(i)) + c_1.*t_vec(i) + c_2;
    else
        opt_pos_vec(i) = v_mp*(t_vec(i)-T_rest_to_MP); 
        opt_spd_vec(i) = v_mp;
     %   opt_acc_vec(i) = 0; 
    end
end
 
end

== matlab function HDVPSG_DelayComp_NewRef_RealDrop_case1/ARE_First_Order_Derivative_[1,0,0]6/MATLAB Function ==
  data: U input; Dot_U output; Ts input; u_init input
function Dot_U = buffer(U, Ts, u_init)
    N = 12;
    %Ts = 0.01;
    persistent y;
    if isempty(y)
        y=u_init*ones(N+1,1);%m/s
    end

    y = [U;y(1:end-1)];
    T = Ts*N;
    P = zeros(1,N+1);
    P_alpha = P;
    for k = 1:N+1
        tao_k = (k-1)*Ts;
        P(k) = T-2*tao_k;
        if((k==1)||(k==N+1))
            P_alpha(k) = P(k)*Ts/2;
        else
            P_alpha(k) = P(k)*Ts;
        end
    end
    
    Dot_U = P_alpha*y*6/(T^3);

end

== matlab function HDVPSG_DelayComp_NewRef_RealDrop_case1/PSG3_control_withPDR_compen/MATLAB Function ==
  data: REALWORLD_DIST output; X_Ego input; Rho_delta_d_adpt output; Y_Ego input; X_Front input; Y_Front input; DELTA_D_MIN input; Rho_delta_dMAX input
function [REALWORLD_DIST, Rho_delta_d_adpt] = Adaptive_Rho_delta_d(X_Ego, Y_Ego, X_Front, Y_Front, DELTA_D_MIN, Rho_delta_dMAX)
    REALWORLD_DIST = sqrt((X_Ego - X_Front)^2 + (Y_Ego - Y_Front)^2); % The virtual leading car may be in another lane: So far away from the ego_car

    if REALWORLD_DIST>2*DELTA_D_MIN  %  This is determined by the road geometry
        Rho_delta_d_adpt = 0; % Disable 
    elseif REALWORLD_DIST>DELTA_D_MIN
        Rho_delta_d_adpt = -Rho_delta_dMAX/DELTA_D_MIN*REALWORLD_DIST + 2*Rho_delta_dMAX;   % linear adaptive gain
    else
        Rho_delta_d_adpt = Rho_delta_dMAX;
    end
    
end

== matlab function HDVPSG_DelayComp_NewRef_RealDrop_case1/PSG2_control_withPDR_compen/MATLAB Function2 ==
  data: Recv input; Lost_Step output
function Lost_Step = fcn(Recv)
  persistent NUM;
  if isempty(NUM)
      NUM =0;
  end
      
  if Recv == 0
      NUM = NUM +1;
  else
      NUM = 0;
  end
  Lost_Step = NUM;
end

== matlab function HDVPSG_DelayComp_NewRef_RealDrop_case1/PSG3_control_withPDR_compen/Subsystem2/MATLAB Function3 ==
  data: Lost_Step input; delta_d_pre_freeze_if_lost input; delta_d_measure input; delta_d_MPC output
function delta_d_MPC  = fcn(Lost_Step, delta_d_pre_freeze_if_lost, delta_d_measure)
    if Lost_Step == 0
        delta_d_MPC   = delta_d_measure;
        %delta_d_dot_enhanced = delta_d_dot_measure;
    else
        delta_d_MPC   = delta_d_pre_freeze_if_lost(Lost_Step);
        %delta_d_dot_enhanced = delta_d_dot_pre_freeze_if_lost(Lost_Step); 
    end
end

== matlab function HDVPSG_DelayComp_NewRef_RealDrop_case1/PSG2_control_withPDR_compen/PRE_OPT_Pos ==
  data: alpha_pre input; opt_pos_pre output; opt_spd_pre output; beta_pre input; c_1_pre input; c_2_pre input; c_3_pre input; c_4_pre input; v_mp input; T_all_to_MP_pre input; t_aft_trigger_pre input; opt_pos_pre_vec output; opt_spd_pre_vec output
function [opt_pos_pre, opt_spd_pre, opt_pos_pre_vec, opt_spd_pre_vec] = Opt_Pos_Ref_Pre(alpha_pre, beta_pre, c_1_pre, c_2_pre, c_3_pre, c_4_pre, v_mp, T_all_to_MP_pre, t_aft_trigger_pre)
Np              = 20;
opt_pos_pre_vec = zeros(1, Np+1);
opt_spd_pre_vec = zeros(1, Np+1);
%opt_acc_vec = zeros(1, Np+1);

Ts    = 0.01;
 % t = min(t, T_rest_to_MP);
  t_vec = t_aft_trigger_pre + (1:(Np+1))*Ts;
 
 if t_aft_trigger_pre <= T_all_to_MP_pre
     opt_pos_pre = -alpha_pre.*exp(t_aft_trigger_pre) + beta_pre.*exp(-t_aft_trigger_pre) + 1/6.*c_1_pre.*t_aft_trigger_pre.^3 + c_2_pre./2.*t_aft_trigger_pre.^2 + c_3_pre.*t_aft_trigger_pre + c_4_pre;
     opt_spd_pre = -alpha_pre.*exp(t_aft_trigger_pre) - beta_pre.*exp(-t_aft_trigger_pre) + 1/2.*c_1_pre.*t_aft_trigger_pre.^2 + c_2_pre.*t_aft_trigger_pre + c_3_pre;
 else
     opt_pos_pre = v_mp*(t_aft_trigger_pre-T_all_to_MP_pre);
     opt_spd_pre = v_mp;
 end
 
for i = 1:Np+1
    if t_vec(i)<=T_all_to_MP_pre
        opt_pos_pre_vec(i) = -alpha_pre.*exp(t_vec(i)) + beta_pre.*exp(-t_vec(i)) + 1/6.*c_1_pre.*t_vec(i).^3 + c_2_pre./2.*t_vec(i).^2 + c_3_pre.*t_vec(i) + c_4_pre;
        opt_spd_pre_vec(i) = -alpha_pre.*exp(t_vec(i)) - beta_pre.*exp(-t_vec(i)) + 1/2.*c_1_pre.*t_vec(i).^2 + c_2_pre.*t_vec(i)       + c_3_pre;
      %  opt_acc_vec(i) = -alpha.*exp(t_vec(i)) + beta.*exp(-t_vec(i)) + c_1.*t_vec(i) + c_2;
    else
        opt_pos_pre_vec(i) = v_mp*(t_vec(i)-T_all_to_MP_pre); 
        opt_spd_pre_vec(i) = v_mp;
     %   opt_acc_vec(i) = 0; 
    end
end
 
end

== matlab function HDVPSG_DelayComp_NewRef_RealDrop_case1/PSG2_control_withPDR_compen/SELF_Optimal_Control_Reference ==
  data: opt_spd output; L_ctz input; opt_pos output; v_ini input; a_ini input; T_all_to_MP input; v_mp input; t_aft_trigger input; opt_acc output; opt_pos_vec output; opt_spd_vec output; alpha output; beta output; c_1 output; c_2 output; c_3 output; c_4 output
function [opt_spd, opt_pos, opt_acc, opt_pos_vec, opt_spd_vec, alpha, beta, c_1, c_2, c_3, c_4] = Opt_Ref(L_ctz, v_ini, a_ini, T_all_to_MP, v_mp, t_aft_trigger)
Np          = 20;
opt_pos_vec = zeros(1, Np+1);
opt_spd_vec = zeros(1, Np+1);
%opt_acc_vec = zeros(1, Np+1);

Ts    = 0.01;
L_ctz = -L_ctz;

alpha = -(12*v_mp - 12*v_ini - 12*L_ctz - 6*T_all_to_MP*a_ini - 12*T_all_to_MP*v_mp + 6*T_all_to_MP*L_ctz + 2*T_all_to_MP^2*a_ini + 2*T_all_to_MP^2*v_ini + 4*T_all_to_MP^2*v_mp + 12*v_ini*exp(-T_all_to_MP) - 12*v_mp*exp(-T_all_to_MP) + 12*L_ctz*exp(-T_all_to_MP) + 6*T_all_to_MP*a_ini*exp(-T_all_to_MP) + 12*T_all_to_MP*v_ini*exp(-T_all_to_MP) + 6*T_all_to_MP*L_ctz*exp(-T_all_to_MP) + 4*T_all_to_MP^2*a_ini*exp(-T_all_to_MP) + T_all_to_MP^3*a_ini*exp(-T_all_to_MP) + 4*T_all_to_MP^2*v_ini*exp(-T_all_to_MP) + 2*T_all_to_MP^2*v_mp*exp(-T_all_to_MP))/(24*exp(-T_all_to_MP) + 24*exp(T_all_to_MP) + 8*T_all_to_MP^2*exp(-T_all_to_MP) + T_all_to_MP^3*exp(-T_all_to_MP) - 24*T_all_to_MP*exp(T_all_to_MP) + 8*T_all_to_MP^2 + 24*T_all_to_MP*exp(-T_all_to_MP) + 8*T_all_to_MP^2*exp(T_all_to_MP) - T_all_to_MP^3*exp(T_all_to_MP) - 48);

beta  = -(12*v_mp - 12*v_ini + 12*L_ctz - 6*T_all_to_MP*a_ini + 12*T_all_to_MP*v_mp + 6*T_all_to_MP*L_ctz - 2*T_all_to_MP^2*a_ini + 2*T_all_to_MP^2*v_ini + 4*T_all_to_MP^2*v_mp + 12*v_ini*exp(T_all_to_MP) - 12*v_mp*exp(T_all_to_MP) - 12*L_ctz*exp(T_all_to_MP) - 4*T_all_to_MP^2*a_ini*exp(T_all_to_MP) + T_all_to_MP^3*a_ini*exp(T_all_to_MP) + 4*T_all_to_MP^2*v_ini*exp(T_all_to_MP) + 2*T_all_to_MP^2*v_mp*exp(T_all_to_MP) + 6*T_all_to_MP*a_ini*exp(T_all_to_MP) - 12*T_all_to_MP*v_ini*exp(T_all_to_MP) + 6*T_all_to_MP*L_ctz*exp(T_all_to_MP))/(24*exp(-T_all_to_MP) + 24*exp(T_all_to_MP) + 8*T_all_to_MP^2*exp(-T_all_to_MP) + T_all_to_MP^3*exp(-T_all_to_MP) - 24*T_all_to_MP*exp(T_all_to_MP) + 8*T_all_to_MP^2 + 24*T_all_to_MP*exp(-T_all_to_MP) + 8*T_all_to_MP^2*exp(T_all_to_MP) - T_all_to_MP^3*exp(T_all_to_MP) - 48);

  c_1 = -(6*(8*L_ctz - 8*a_ini + 4*T_all_to_MP*v_ini + 4*T_all_to_MP*v_mp + 2*T_all_to_MP^2*a_ini + 4*a_ini*exp(T_all_to_MP) - 4*L_ctz*exp(T_all_to_MP) + 4*a_ini*exp(-T_all_to_MP) - 4*L_ctz*exp(-T_all_to_MP) + 4*T_all_to_MP*a_ini*exp(-T_all_to_MP) + T_all_to_MP^2*a_ini*exp(T_all_to_MP) - 2*T_all_to_MP*v_ini*exp(-T_all_to_MP) + T_all_to_MP^2*v_ini*exp(T_all_to_MP) - 2*T_all_to_MP*v_mp*exp(-T_all_to_MP) + T_all_to_MP^2*v_mp*exp(T_all_to_MP) - 2*T_all_to_MP*L_ctz*exp(-T_all_to_MP) + T_all_to_MP^2*a_ini*exp(-T_all_to_MP) - T_all_to_MP^2*v_ini*exp(-T_all_to_MP) - T_all_to_MP^2*v_mp*exp(-T_all_to_MP) - 4*T_all_to_MP*a_ini*exp(T_all_to_MP) - 2*T_all_to_MP*v_ini*exp(T_all_to_MP) - 2*T_all_to_MP*v_mp*exp(T_all_to_MP) + 2*T_all_to_MP*L_ctz*exp(T_all_to_MP)))/(T_all_to_MP*(24*exp(-T_all_to_MP) + 24*exp(T_all_to_MP) + 8*T_all_to_MP^2*exp(-T_all_to_MP) + T_all_to_MP^3*exp(-T_all_to_MP) - 24*T_all_to_MP*exp(T_all_to_MP) + 8*T_all_to_MP^2 + 24*T_all_to_MP*exp(-T_all_to_MP) + 8*T_all_to_MP^2*exp(T_all_to_MP) - T_all_to_MP^3*exp(T_all_to_MP) - 48)); 
  
  c_2 = (2*(12*L_ctz - 24*a_ini + 12*T_all_to_MP*v_mp + 2*T_all_to_MP^2*a_ini + 12*a_ini*exp(T_all_to_MP) + 6*v_ini*exp(T_all_to_MP) - 6*v_mp*exp(T_all_to_MP) - 6*L_ctz*exp(T_all_to_MP) + 12*a_ini*exp(-T_all_to_MP) - 6*v_ini*exp(-T_all_to_MP) + 6*v_mp*exp(-T_all_to_MP) - 6*L_ctz*exp(-T_all_to_MP) + 9*T_all_to_MP*a_ini*exp(-T_all_to_MP) + 2*T_all_to_MP^2*a_ini*exp(T_all_to_MP) - 6*T_all_to_MP*v_ini*exp(-T_all_to_MP) + 2*T_all_to_MP^2*v_ini*exp(T_all_to_MP) + T_all_to_MP^2*v_mp*exp(T_all_to_MP) - 3*T_all_to_MP*L_ctz*exp(-T_all_to_MP) + 2*T_all_to_MP^2*a_ini*exp(-T_all_to_MP) - 2*T_all_to_MP^2*v_ini*exp(-T_all_to_MP) - T_all_to_MP^2*v_mp*exp(-T_all_to_MP) - 9*T_all_to_MP*a_ini*exp(T_all_to_MP) - 6*T_all_to_MP*v_ini*exp(T_all_to_MP) + 3*T_all_to_MP*L_ctz*exp(T_all_to_MP)))/(24*exp(-T_all_to_MP) + 24*exp(T_all_to_MP) + 8*T_all_to_MP^2*exp(-T_all_to_MP) + T_all_to_MP^3*exp(-T_all_to_MP) - 24*T_all_to_MP*exp(T_all_to_MP) + 8*T_all_to_MP^2 + 24*T_all_to_MP*exp(-T_all_to_MP) + 8*T_all_to_MP^2*exp(T_all_to_MP) - T_all_to_MP^3*exp(T_all_to_MP) - 48); 
  
  c_3 = -(24*v_ini + 24*v_mp - 12*T_all_to_MP*a_ini + 12*T_all_to_MP*L_ctz - 4*T_all_to_MP^2*v_ini + 8*T_all_to_MP^2*v_mp - 12*v_ini*exp(T_all_to_MP) - 12*v_mp*exp(T_all_to_MP) - 12*L_ctz*exp(T_all_to_MP) - 12*v_ini*exp(-T_all_to_MP) - 12*v_mp*exp(-T_all_to_MP) + 12*L_ctz*exp(-T_all_to_MP) + 6*T_all_to_MP*a_ini*exp(-T_all_to_MP) - 4*T_all_to_MP^2*a_ini*exp(T_all_to_MP) + T_all_to_MP^3*a_ini*exp(T_all_to_MP) - 12*T_all_to_MP*v_ini*exp(-T_all_to_MP) - 4*T_all_to_MP^2*v_ini*exp(T_all_to_MP) + T_all_to_MP^3*v_ini*exp(T_all_to_MP) + 2*T_all_to_MP^2*v_mp*exp(T_all_to_MP) + 6*T_all_to_MP*L_ctz*exp(-T_all_to_MP) + 4*T_all_to_MP^2*a_ini*exp(-T_all_to_MP) + T_all_to_MP^3*a_ini*exp(-T_all_to_MP) - 4*T_all_to_MP^2*v_ini*exp(-T_all_to_MP) - T_all_to_MP^3*v_ini*exp(-T_all_to_MP) + 2*T_all_to_MP^2*v_mp*exp(-T_all_to_MP) + 6*T_all_to_MP*a_ini*exp(T_all_to_MP) + 12*T_all_to_MP*v_ini*exp(T_all_to_MP) + 6*T_all_to_MP*L_ctz*exp(T_all_to_MP))/(24*exp(-T_all_to_MP) + 24*exp(T_all_to_MP) + 8*T_all_to_MP^2*exp(-T_all_to_MP) + T_all_to_MP^3*exp(-T_all_to_MP) - 24*T_all_to_MP*exp(T_all_to_MP) + 8*T_all_to_MP^2 + 24*T_all_to_MP*exp(-T_all_to_MP) + 8*T_all_to_MP^2*exp(T_all_to_MP) - T_all_to_MP^3*exp(T_all_to_MP) - 48); 
  
  c_4 = -(24*L_ctz - 24*T_all_to_MP*v_mp + 4*T_all_to_MP^2*a_ini - 8*T_all_to_MP^2*L_ctz - 12*v_ini*exp(T_all_to_MP) + 12*v_mp*exp(T_all_to_MP) - 12*L_ctz*exp(T_all_to_MP) + 12*v_ini*exp(-T_all_to_MP) - 12*v_mp*exp(-T_all_to_MP) - 12*L_ctz*exp(-T_all_to_MP) + 6*T_all_to_MP*a_ini*exp(-T_all_to_MP) + 4*T_all_to_MP^2*a_ini*exp(T_all_to_MP) - T_all_to_MP^3*a_ini*exp(T_all_to_MP) + 12*T_all_to_MP*v_ini*exp(-T_all_to_MP) - 4*T_all_to_MP^2*v_ini*exp(T_all_to_MP) - 2*T_all_to_MP^2*v_mp*exp(T_all_to_MP) - 18*T_all_to_MP*L_ctz*exp(-T_all_to_MP) - 8*T_all_to_MP^2*L_ctz*exp(T_all_to_MP) + T_all_to_MP^3*L_ctz*exp(T_all_to_MP) + 4*T_all_to_MP^2*a_ini*exp(-T_all_to_MP) + T_all_to_MP^3*a_ini*exp(-T_all_to_MP) + 4*T_all_to_MP^2*v_ini*exp(-T_all_to_MP) + 2*T_all_to_MP^2*v_mp*exp(-T_all_to_MP) - 8*T_all_to_MP^2*L_ctz*exp(-T_all_to_MP) - T_all_to_MP^3*L_ctz*exp(-T_all_to_MP) - 6*T_all_to_MP*a_ini*exp(T_all_to_MP) + 12*T_all_to_MP*v_ini*exp(T_all_to_MP) + 18*T_all_to_MP*L_ctz*exp(T_all_to_MP))/(24*exp(-T_all_to_MP) + 24*exp(T_all_to_MP) + 8*T_all_to_MP^2*exp(-T_all_to_MP) + T_all_to_MP^3*exp(-T_all_to_MP) - 24*T_all_to_MP*exp(T_all_to_MP) + 8*T_all_to_MP^2 + 24*T_all_to_MP*exp(-T_all_to_MP) + 8*T_all_to_MP^2*exp(T_all_to_MP) - T_all_to_MP^3*exp(T_all_to_MP) - 48);
  
 % t = min(t, T_rest_to_MP);
  t_vec = t_aft_trigger + (1:(Np+1))*Ts;
 
 if t_aft_trigger <= T_all_to_MP
     opt_pos = -alpha.*exp(t_aft_trigger) + beta.*exp(-t_aft_trigger) + 1/6.*c_1.*t_aft_trigger.^3 + c_2./2.*t_aft_trigger.^2 + c_3.*t_aft_trigger + c_4;
     opt_spd = -alpha.*exp(t_aft_trigger) - beta.*exp(-t_aft_trigger) + 1/2.*c_1.*t_aft_trigger.^2 + c_2.*t_aft_trigger + c_3;
     opt_acc = -alpha.*exp(t_aft_trigger) + beta.*exp(-t_aft_trigger) + c_1.*t_aft_trigger + c_2;
 else
     opt_pos = v_mp*(t_aft_trigger-T_all_to_MP);
     opt_spd = v_mp;
     opt_acc = 0;
 end
 
for i = 1:Np+1
    if t_vec(i)<=T_all_to_MP
        opt_pos_vec(i) = -alpha.*exp(t_vec(i)) + beta.*exp(-t_vec(i)) + 1/6.*c_1.*t_vec(i).^3 + c_2./2.*t_vec(i).^2 + c_3.*t_vec(i) + c_4;
        opt_spd_vec(i) = -alpha.*exp(t_vec(i)) - beta.*exp(-t_vec(i)) + 1/2.*c_1.*t_vec(i).^2 + c_2.*t_vec(i)       + c_3;
      %  opt_acc_vec(i) = -alpha.*exp(t_vec(i)) + beta.*exp(-t_vec(i)) + c_1.*t_vec(i) + c_2;
    else
        opt_pos_vec(i) = v_mp*(t_vec(i)-T_all_to_MP); 
        opt_spd_vec(i) = v_mp;
     %   opt_acc_vec(i) = 0; 
    end
end
 
end

== matlab function HDVPSG_DelayComp_NewRef_RealDrop_case1/PSG2_control_withPDR_compen/States_update2 ==
  data: x0 output; delta_d input; delta_d_dot input
function x0 = Init(delta_d, delta_d_dot)
    x0 = [delta_d;
          delta_d_dot];
end

== matlab function HDVPSG_DelayComp_NewRef_RealDrop_case1/PSG2_control_withPDR_compen/Subsystem17/Poly_coefficient ==
  data: a_0 output; delta_d0 input; a_1 output; a_2 output; delta_dTCC input; delta_v0 input; Tend input; a_3 output
function [a_0, a_1, a_2, a_3] = poly_4_coefficient(delta_d0, delta_dTCC, delta_v0, Tend)
% With conditions:
% delta_d_0 given,            delta_v_0 given 
% delta_d_Tend = delta_d_TTC, delta_v_Tend = 0

% delta_dr(t) = a0 + a1*t + a2*t^2 + a3*t^3
    a_0 = delta_d0;
    a_1 = delta_v0;
    a_2 = -(3*delta_d0 - 3*delta_dTCC + 2*Tend*delta_v0)/Tend^2;
    a_3 = (2*delta_d0 - 2*delta_dTCC + Tend*delta_v0)/Tend^3;
end

== matlab function HDVPSG_DelayComp_NewRef_RealDrop_case1/Subsystem1/Subsystem4/MATLAB Function ==
  data: distMP input; HighTRFC output
function HighTRFC = fcn(distMP)
    if distMP<=150 && distMP>=120
        HighTRFC = 0; % iced road 
    else 
        HighTRFC = 1;
    end 
end

== matlab function HDVPSG_DelayComp_NewRef_RealDrop_case1/Subsystem1/Subsystem5/MATLAB Function ==
  data: distMP input; HighTRFC output
function HighTRFC = fcn(distMP)
    if distMP<=150 && distMP>=120
        HighTRFC = 0; % iced road 
    else 
        HighTRFC = 1;
    end 
end

== matlab function HDVPSG_DelayComp_NewRef_RealDrop_case1/Subsystem1/Subsystem6/MATLAB Function ==
  data: distMP input; HighTRFC output
function HighTRFC = fcn(distMP)
    if distMP<=150 && distMP>=120
        HighTRFC = 0; % iced road 
    else 
        HighTRFC = 1;
    end 
end

== matlab function HDVPSG_DelayComp_NewRef_RealDrop_case1/Subsystem1/Subsystem7/MATLAB Function ==
  data: distMP input; HighTRFC output
function HighTRFC = fcn(distMP)
    if distMP<=150 && distMP>=120
        HighTRFC = 0; % iced road 
    else 
        HighTRFC = 1;
    end 
end

== matlab function HDVPSG_DelayComp_NewRef_RealDrop_case1/Subsystem2/Subsystem4/MATLAB Function ==
  data: distMP input; HighTRFC output
function HighTRFC = fcn(distMP)
    if distMP<=150 && distMP>=120
        HighTRFC = 0; % iced road 
    else 
        HighTRFC = 1;
    end 
end

== matlab function HDVPSG_DelayComp_NewRef_RealDrop_case1/Subsystem2/Subsystem5/MATLAB Function ==
  data: distMP input; HighTRFC output
function HighTRFC = fcn(distMP)
    if distMP<=150 && distMP>=120
        HighTRFC = 0; % iced road 
    else 
        HighTRFC = 1;
    end 
end

== matlab function HDVPSG_DelayComp_NewRef_RealDrop_case1/Subsystem29/Subsystem4/MATLAB Function ==
  data: distMP input; HighTRFC output
function HighTRFC = fcn(distMP)
    if distMP<=150 && distMP>=120
        HighTRFC = 0; % iced road 
    else 
        HighTRFC = 1;
    end 
end

== matlab function HDVPSG_DelayComp_NewRef_RealDrop_case1/Subsystem29/Subsystem5/MATLAB Function ==
  data: distMP input; HighTRFC output
function HighTRFC = fcn(distMP)
    if distMP<=150 && distMP>=120
        HighTRFC = 0; % iced road 
    else 
        HighTRFC = 1;
    end 
end

== matlab function HDVPSG_DelayComp_NewRef_RealDrop_case1/Subsystem29/Subsystem6/MATLAB Function ==
  data: distMP input; HighTRFC output
function HighTRFC = fcn(distMP)
    if distMP<=150 && distMP>=120
        HighTRFC = 0; % iced road 
    else 
        HighTRFC = 1;
    end 
end

== matlab function HDVPSG_DelayComp_NewRef_RealDrop_case1/PSG2_control_withPDR_compen/Subsystem18/Ref ==
  data: delta_dr output; a_0 input; delta_dr_dot output; a_1 input; a_2 input; a_3 input; t_sumo input
function [delta_dr, delta_dr_dot] = poly_4_reference(a_0, a_1, a_2, a_3, t_sumo)
    delta_dr     = a_0 + a_1*t_sumo + a_2*t_sumo^2 + a_3*t_sumo^3;
    delta_dr_dot =       a_1        + 2*a_2*t_sumo + 3*a_3*t_sumo^2;
end

== matlab function HDVPSG_DelayComp_NewRef_RealDrop_case1/PSG2_control_withPDR_compen/Subsystem18/Ref_Pre_Vec ==
  data: delta_dr_Pre_Vec output; a_0 input; delta_dr_dot_Pre_Vec output; a_1 input; a_2 input; a_3 input; t_sumo input
function [delta_dr_Pre_Vec, delta_dr_dot_Pre_Vec] = poly_4_reference(a_0, a_1, a_2, a_3, t_sumo)
    Ts = 0.01;
    Np = 20;
    
    t_Pre_Vec = t_sumo + (1:Np+1)*Ts;
    
    delta_dr_Pre_Vec     = a_0 + a_1*t_Pre_Vec + a_2*t_Pre_Vec.^2 + a_3*t_Pre_Vec.^3;
    delta_dr_dot_Pre_Vec =       a_1           + 2*a_2*t_Pre_Vec  + 3*a_3*t_Pre_Vec.^2;
end

== matlab function HDVPSG_DelayComp_NewRef_RealDrop_case1/ARE_First_Order_Derivative_[1,0,0]8/MATLAB Function ==
  data: U input; Dot_U output; Ts input; u_init input
function Dot_U = buffer(U, Ts, u_init)
    N = 12;
    %Ts = 0.01;
    persistent y;
    if isempty(y)
        y=u_init*ones(N+1,1);%m/s
    end

    y = [U;y(1:end-1)];
    T = Ts*N;
    P = zeros(1,N+1);
    P_alpha = P;
    for k = 1:N+1
        tao_k = (k-1)*Ts;
        P(k) = T-2*tao_k;
        if((k==1)||(k==N+1))
            P_alpha(k) = P(k)*Ts/2;
        else
            P_alpha(k) = P(k)*Ts;
        end
    end
    
    Dot_U = P_alpha*y*6/(T^3);

end
